simulink model "Pilot_Joystick_All"  (R2014a)
settings: Solver=ode45  StartTime=0.0  StopTime=Inf  RelTol=1e-3
libraries: aerolibanimutils x3, UWAerospaceBlockset_Animation x2
settings Model: Creator=Christopher  LastModifiedBy=Christopher

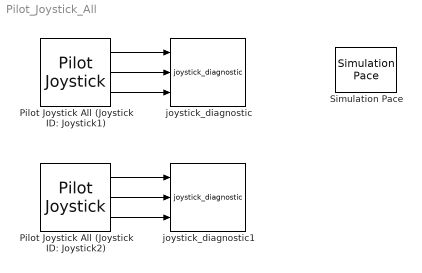
== system Pilot_Joystick_All ==
  Pilot Joystick All (Joystick ID: Joystick1) : aerolibanimutils/Pilot Joystick  JoystickID=Joystick1  OutputConfiguration=AllOutputs  SampleTime=1/30
  Pilot Joystick All (Joystick ID: Joystick2) : aerolibanimutils/Pilot Joystick  JoystickID=Joystick2  OutputConfiguration=AllOutputs  SampleTime=1/30
  Simulation Pace : aerolibanimutils/Simulation Pace  SimulationPace=1  SleepMode=MATLAB Thread  OutputPaceError=off  SampleTime=1/30
      settings: AttributesFormatString=%<SimulationPace> sec/sec
  joystick_diagnostic : UWAerospaceBlockset_Animation/joystick_diagnostic
  joystick_diagnostic1 : UWAerospaceBlockset_Animation/joystick_diagnostic
  wires:
  Pilot Joystick All (Joystick ID: Joystick1)/2 -> joystick_diagnostic/2
  Pilot Joystick All (Joystick ID: Joystick1)/3 -> joystick_diagnostic/3
  Pilot Joystick All (Joystick ID: Joystick1)/1 -> joystick_diagnostic/1
  Pilot Joystick All (Joystick ID: Joystick2)/3 -> joystick_diagnostic1/3
  Pilot Joystick All (Joystick ID: Joystick2)/2 -> joystick_diagnostic1/2
  Pilot Joystick All (Joystick ID: Joystick2)/1 -> joystick_diagnostic1/1
